simulink library "lib_interactive"  (Simulink 4.1.1)
undefined symbols (not defined in the file or in its folder): ALTIAHOME, pause_time
libraries: lib_interactive x1
settings Model: LastModifiedBy=abrooker  ModifiedComment=abrooker -- Tue May 14 11:03:09 2002 -- Version 1.239
settings Model: ModifiedHistory=|
  | abrooker -- Tue May 14 11:03:09 2002 -- Version 1.239
  | 
  | 
  | mokeefe -- Thu Apr 18 08:35:49 2002 -- Version 1.238
  | saving the model:
  | o "without the model browser open"
  | o with only top-level screen visible
  | o with "fit to view" enabled
  | o with "status bar" off and "toolbar" off
  | o with "prompt to update model history with each save" on

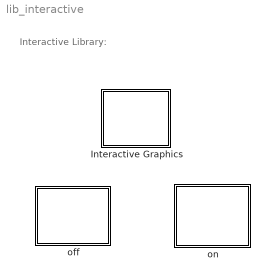
== system lib_interactive ==
  note: Interactive Library:
  Interactive Graphics : Subsystem  BlockChoice=off
      settings: TemplateBlock=self  MemberBlocks=off,on  RTWFcnNameOpts=Auto  RTWFileNameOpts=Auto
  off : Subsystem  Tag=Altia_off  Orientation=up
      settings: RTWFcnNameOpts=Auto  RTWFileNameOpts=Auto
      mask Display: image(imread('results.bmp'))
  on : Subsystem  Tag=Altia_on  Orientation=up
      settings: RTWFcnNameOpts=Auto  RTWFileNameOpts=Auto
      mask Display: image(imread('interactive.bmp'))

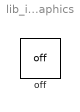
== system lib_interactive/Interactive Graphics ==
  off : lib_interactive/off  Tag=Altia_off  Orientation=up

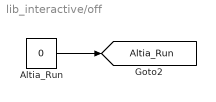
== system lib_interactive/off ==
  Altia_Run : Constant  Value=0
  tag scope: Altia_Run=global
  wires:
  Altia_Run/1 -> [Altia_Run]

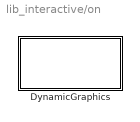
== system lib_interactive/on ==
  DynamicGraphics : Subsystem
      mask init:
      | [fileInfo,resultFile]=getFileInfo;
      | axisLimits=writeAltiaBmps(1,fileInfo);
      | writeAltiaInfoFile(1,fileInfo,resultFile,axisLimits);
      settings: RTWFcnNameOpts=Auto  RTWFileNameOpts=Auto

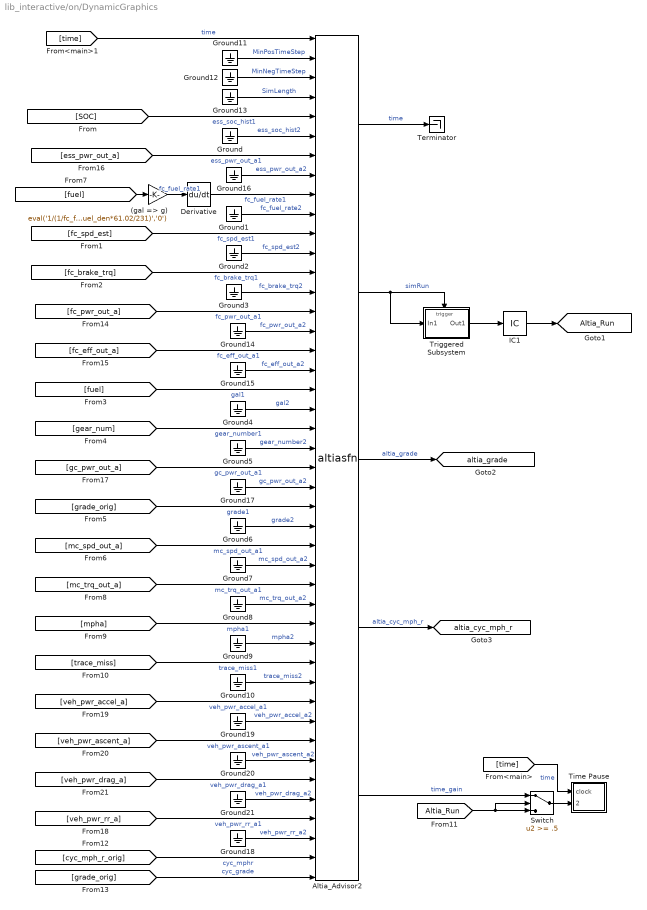
== system lib_interactive/on/DynamicGraphics ==
  (gal => g) : Gain  Gain=eval('1/(1/fc_fuel_den*61.02/231)','0')  Multiplication=Element-wise(K.*u)  SaturateOnIntegerOverflow=on
  Altia_Advisor2 : S-Function  FunctionName=altiasfn  Parameters=NumAltiaSfnInputs,NumAltiaSfnOutputs,ALTIAHOME  PortCounts=[]  SFunctionModules=libsdde.lib user32.lib  mask{NumAltiaSfnInputs=44, NumAltiaSfnOutputs=5}
      mask prompts: NumAltiaSfnInputs "Inputs to Altia S-Function:"; NumAltiaSfnOutputs "Outputs to Altia S-Function:"
      mask help: This block allows you to connect your signals to an Altia Design file. Specify the number of Inputs and Outputs you would like the Altia block to have (each line connected to the block can only be ONE signal wide ... no muxing into the Altia block).
      mask init:
      | altiahome
      settings: OpenFcn=AltiaClk
      mask Help: The first box is the number of inputs to the Altia S-Function.  The second box is the number of ouputs for the Altia S-Function.
      mask Display: disp('A L T I A')
  Derivative : Derivative
  Ground{,1..21} (22 alike) : Ground
  IC1 : InitialCondition  Value=1
  Switch : Switch  Threshold=.5
  Terminator : Terminator
  Time Pause : Subsystem
      settings: RTWFcnNameOpts=Auto  RTWFileNameOpts=Auto
  Triggered Subsystem : Subsystem  TreatAsAtomicUnit=on
      settings: RTWFcnNameOpts=Auto  RTWFileNameOpts=Auto
  tag scope: Altia_Run=global, altia_cyc_mph_r=global, altia_grade=global
  wires:
  Triggered Subsystem/1(Out1) -> IC1/1
  Altia_Advisor2/2 -> Triggered Subsystem/1(In1), Triggered Subsystem/Trigger  "simRun"
  [grade_orig] -> Altia_Advisor2/44  "cyc_grade"
  [cyc_mph_r_orig] -> Altia_Advisor2/43  "cyc_mphr"
  Altia_Advisor2/1 -> Terminator/1  "time"
  Ground11/1 -> Altia_Advisor2/2  "MinPosTimeStep"
  Ground12/1 -> Altia_Advisor2/3  "MinNegTimeStep"
  Ground13/1 -> Altia_Advisor2/4  "SimLength"
  [time] -> Altia_Advisor2/1  "time"
  [SOC] -> Altia_Advisor2/5  "ess_soc_hist1"
  Ground/1 -> Altia_Advisor2/6  "ess_soc_hist2"
  [fuel] -> (gal => g)/1
  Ground1/1 -> Altia_Advisor2/10  "fc_fuel_rate2"
  [fc_spd_est] -> Altia_Advisor2/11  "fc_spd_est1"
  Ground2/1 -> Altia_Advisor2/12  "fc_spd_est2"
  [fc_brake_trq] -> Altia_Advisor2/13  "fc_brake_trq1"
  Ground3/1 -> Altia_Advisor2/14  "fc_brake_trq2"
  [fuel] -> Altia_Advisor2/19  "gal1"
  Ground4/1 -> Altia_Advisor2/20  "gal2"
  [gear_num] -> Altia_Advisor2/21  "gear_number1"
  Ground5/1 -> Altia_Advisor2/22  "gear_number2"
  [grade_orig] -> Altia_Advisor2/25  "grade1"
  Ground6/1 -> Altia_Advisor2/26  "grade2"
  [mc_spd_out_a] -> Altia_Advisor2/27  "mc_spd_out_a1"
  Ground7/1 -> Altia_Advisor2/28  "mc_spd_out_a2"
  [mc_trq_out_a] -> Altia_Advisor2/29  "mc_trq_out_a1"
  Ground8/1 -> Altia_Advisor2/30  "mc_trq_out_a2"
  [mpha] -> Altia_Advisor2/31  "mpha1"
  Ground9/1 -> Altia_Advisor2/32  "mpha2"
  [trace_miss] -> Altia_Advisor2/33  "trace_miss1"
  Ground10/1 -> Altia_Advisor2/34  "trace_miss2"
  Altia_Advisor2/3 -> [altia_grade]  "altia_grade"
  Altia_Advisor2/4 -> [altia_cyc_mph_r]  "altia_cyc_mph_r"
  Altia_Advisor2/5 -> Switch/1  "time_gain"
  IC1/1 -> [Altia_Run]
  [time] -> Time Pause/1(clock)  "time"
  Switch/1 -> Time Pause/2(time_gain)
  [Altia_Run] -> Switch/3, Switch/2
  (gal => g)/1 -> Derivative/1  "fc_fuel_rate1"
  Derivative/1 -> Altia_Advisor2/9  "fc_fuel_rate1"
  [fc_pwr_out_a] -> Altia_Advisor2/15  "fc_pwr_out_a1"
  Ground14/1 -> Altia_Advisor2/16  "fc_pwr_out_a2"
  [fc_eff_out_a] -> Altia_Advisor2/17  "fc_eff_out_a1"
  Ground15/1 -> Altia_Advisor2/18  "fc_eff_out_a2"
  [ess_pwr_out_a] -> Altia_Advisor2/7  "ess_pwr_out_a1"
  Ground16/1 -> Altia_Advisor2/8  "ess_pwr_out_a2"
  [gc_pwr_out_a] -> Altia_Advisor2/23  "gc_pwr_out_a1"
  Ground17/1 -> Altia_Advisor2/24  "gc_pwr_out_a2"
  [veh_pwr_accel_a] -> Altia_Advisor2/35  "veh_pwr_accel_a1"
  Ground19/1 -> Altia_Advisor2/36  "veh_pwr_accel_a2"
  [veh_pwr_ascent_a] -> Altia_Advisor2/37  "veh_pwr_ascent_a1"
  Ground20/1 -> Altia_Advisor2/38  "veh_pwr_ascent_a2"
  [veh_pwr_drag_a] -> Altia_Advisor2/39  "veh_pwr_drag_a1"
  Ground21/1 -> Altia_Advisor2/40  "veh_pwr_drag_a2"
  [veh_pwr_rr_a] -> Altia_Advisor2/41  "veh_pwr_rr_a1"
  Ground18/1 -> Altia_Advisor2/42  "veh_pwr_rr_a2"

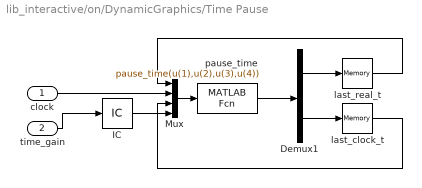
== system lib_interactive/on/DynamicGraphics/Time Pause ==
  clock : Inport  Port=1  LatchInput=off
  time_gain : Inport  Port=2  LatchInput=off
  Demux1 : Demux  Outputs=2  BusSelectionMode=off
  IC : InitialCondition  Value=1
  Mux : Mux  Inputs=4
  last_clock_t : Memory  X0=0  InheritSampleTime=off
      settings: RTWStateStorageClass=Auto
  last_real_t : Memory  X0=0  InheritSampleTime=off
      settings: RTWStateStorageClass=Auto
  pause_time : MATLABFcn  MATLABFcn=pause_time(u(1),u(2),u(3),u(4))  OutputDimensions=2  OutputSignalType=auto  Output1D=on
  wires:
  IC/1 -> Mux/4
  time_gain/1 -> IC/1
  last_real_t/1 -> Mux/1
  last_clock_t/1 -> Mux/3
  Demux1/2 -> last_clock_t/1
  Demux1/1 -> last_real_t/1
  clock/1 -> Mux/2
  pause_time/1 -> Demux1/1
  Mux/1 -> pause_time/1

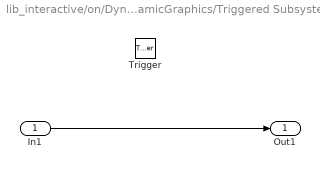
== system lib_interactive/on/DynamicGraphics/Triggered Subsystem ==
  In1 : Inport  Port=1  LatchInput=off
  Trigger : TriggerPort  TriggerType=falling  OutputDataType=auto
  Out1 : Outport  Port=1  InitialOutput=1
  wires:
  In1/1 -> Out1/1
